simulink model "sampleModel1726"  (R2023a)
settings: Solver=VariableStepAuto  StartTime=0.0  StopTime=10.0  RelTol=1e-3
libraries: hdlsllib x4, simulink x2
settings Model: Creator=user1  LastModifiedBy=user1

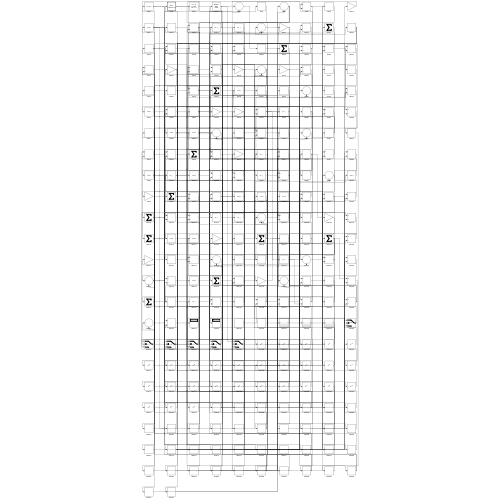
[thumbnail: Simulink's stored preview of the top-level diagram]
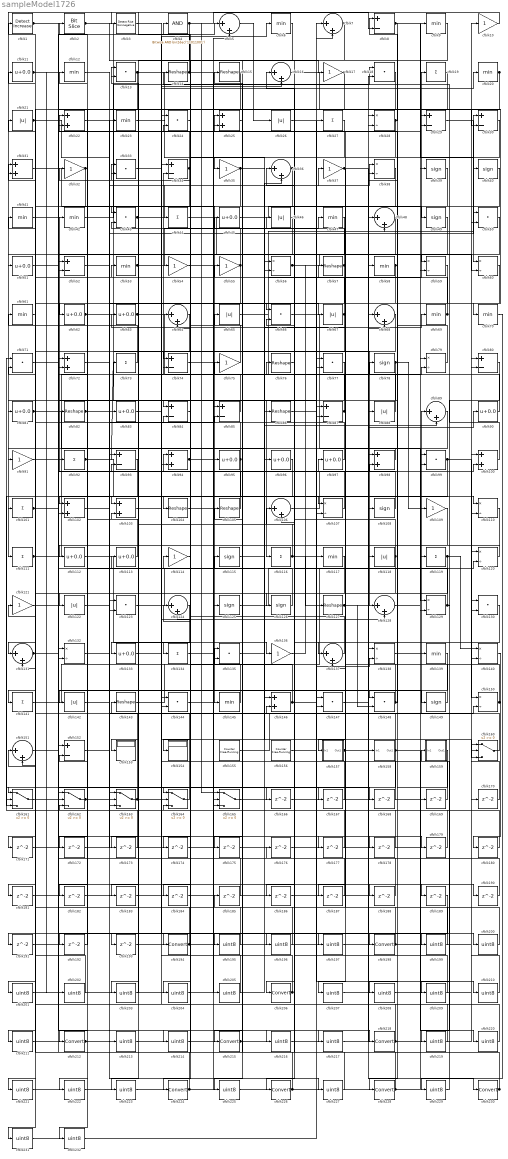
== system sampleModel1726 ==
  cfblk1 : simulink/Logic and Bit Operations/Detect Increase  vinit=0.0  OutDataTypeStr=boolean
      settings: LibrarySourceBlock=|
      | hdlsllib/Logic and Bit
      | Operations/Detect
      | Increase
  cfblk{10,17,32,35,37,54..55,75,91,109,114,121,136} (13 alike) : Gain
  cfblk{22,25,31,72,94,98,100,102..103,146} (10 alike) : Sum
  cfblk{19,27,44,73,92,101,111,116,119,134,141} (11 alike) : Sum  Inputs=+
  cfblk{14..15,57,76,82,86,104..105,127,143} (10 alike) : Reshape
  cfblk{5,7,16,36,48,64,68,89,106,124,128,131,137,151} (14 alike) : Sum  Inputs=|++
  cfblk{28,38,56,59..60,79,107,110,120,129,132,138,140,150} (14 alike) : Product  Inputs=*/  RndMeth=Zero  SaturateOnIntegerOverflow=on
  cfblk{39..40,49,78,108,115,125..126,149} (9 alike) : Signum
  cfblk{11,45,51,62..63,81,83,90,95..97,112..113,133} (14 alike) : Bias  Bias=0.0  SaturateOnIntegerOverflow=off
  cfblk{6,9,12,20,23,41..42,47,53,58,61,69..70,117,139,145} (16 alike) : MinMax
  cfblk{21,26,46,65,67,88,118,122,142} (9 alike) : Abs  SaturateOnIntegerOverflow=off
  cfblk{13,18,24,33,43,50,66,71,77,99,123,130,135,144,147..148} (16 alike) : DotProduct  OutDataTypeStr=Inherit: Inherit via internal rule
  cfblk{8,29..30,34,52,74,80,84..85,87,93,152} (12 alike) : Sum  Inputs=+-
  cfblk153 : Display
  cfblk154 : Display
  cfblk155 : hdlsllib/Sources/Counter Free-Running  NumBits=16  tsamp=-1
  cfblk156 : hdlsllib/Sources/Counter Free-Running  NumBits=16  tsamp=-1
  cfblk157 : Subsystem
      settings: LibrarySourceBlock=|
      | hdlsllib/Ports &
      | Subsystems/Subsystem
  cfblk158 : Subsystem
      settings: LibrarySourceBlock=|
      | hdlsllib/Ports &
      | Subsystems/Subsystem
  cfblk159 : Subsystem
      settings: LibrarySourceBlock=|
      | hdlsllib/Ports &
      | Subsystems/Subsystem
  cfblk{160..165} (6 alike) : Switch  SaturateOnIntegerOverflow=off  InputSameDT=off
  cfblk{166..193} (28 alike) : Delay  SampleTime=1
  cfblk{194,198,206,212,215,218,224,226,228,230} (10 alike) : DataTypeConversion  SaturateOnIntegerOverflow=off  RndMeth=Floor
  cfblk{195..197,199..205,207..211,213..214,216..217,219..223,225,227,229,231..232} (29 alike) : DataTypeConversion  OutDataTypeStr=uint8  SaturateOnIntegerOverflow=off  RndMeth=Floor
  cfblk2 : hdlsllib/Logic and Bit Operations/Bit Slice  lidx=7  ridx=0
  cfblk3 : hdlsllib/Logic and Bit Operations/Detect Rise Nonnegative  vinit=0  OutDataTypeStr=boolean
  cfblk4 : simulink/Logic and Bit Operations/Bitwise Operator  logicop=AND  UseBitMask=on  BitMask=bin2dec('11011001')  BitMaskRealWorld=Stored Integer
      settings: LibrarySourceBlock=|
      | hdlsllib/Logic and Bit
      | Operations/Bitwise
      | Operator
  wires:
  cfblk5/1 -> cfblk26/1
  cfblk119/1 -> cfblk140/1, cfblk126/1, cfblk137/2, cfblk131/1
  cfblk95/1 -> cfblk42/1, cfblk165/2
  cfblk2/1 -> cfblk116/1, cfblk17/1
  cfblk14/1 -> cfblk111/1, cfblk110/1
  cfblk36/1 -> cfblk122/1, cfblk125/1
  cfblk92/1 -> cfblk73/1, cfblk158/1(In1)
  cfblk107/1 -> cfblk72/1
  cfblk76/1 -> cfblk226/1
  cfblk63/1 -> cfblk30/1, cfblk16/2, cfblk160/3
  cfblk16/1 -> cfblk70/1
  cfblk62/1 -> cfblk128/1, cfblk50/1
  cfblk123/1 -> cfblk36/2
  cfblk31/1 -> cfblk145/1
  cfblk29/1 -> cfblk60/1
  cfblk126/1 -> cfblk2/1
  cfblk11/1 -> cfblk30/2, cfblk87/2, cfblk189/1, cfblk202/1
  cfblk155/1 -> cfblk89/1
  cfblk71/1 -> cfblk5/1
  cfblk112/1 -> cfblk136/1
  cfblk149/1 -> cfblk94/1
  cfblk41/1 -> cfblk60/2
  cfblk150/1 -> cfblk55/1, cfblk25/2
  cfblk147/1 -> cfblk230/1
  cfblk7/1 -> cfblk84/1, cfblk104/1, cfblk223/1
  cfblk105/1 -> cfblk53/1
  cfblk68/1 -> cfblk215/1
  cfblk135/1 -> cfblk89/2
  cfblk152/1 -> cfblk198/1
  cfblk158/1(Out1) -> cfblk143/1, cfblk161/3, cfblk220/1
  cfblk42/1 -> cfblk18/1
  cfblk111/1 -> cfblk34/2, cfblk98/2
  cfblk43/1 -> cfblk37/1, cfblk165/3
  cfblk30/1 -> cfblk35/1
  cfblk78/1 -> cfblk134/1, cfblk109/1
  cfblk27/1 -> cfblk224/1
  cfblk136/1 -> cfblk117/1
  cfblk65/1 -> cfblk19/1
  cfblk113/1 -> cfblk52/1
  cfblk106/1 -> cfblk10/1
  cfblk57/1 -> cfblk141/1, cfblk24/2
  cfblk32/1 -> cfblk171/1, cfblk172/1
  cfblk35/1 -> cfblk154/1, cfblk160/2
  cfblk67/1 -> cfblk163/3, cfblk81/1, cfblk31/2
  cfblk17/1 -> cfblk102/1, cfblk232/1
  cfblk13/1 -> cfblk56/2, cfblk192/1
  cfblk141/1 -> cfblk28/1
  cfblk45/1 -> cfblk49/1
  cfblk75/1 -> cfblk32/1
  cfblk12/1 -> cfblk194/1
  cfblk90/1 -> cfblk33/1
  cfblk69/1 -> cfblk15/1, cfblk11/1
  cfblk97/1 -> cfblk41/1
  cfblk98/1 -> cfblk91/1
  cfblk118/1 -> cfblk63/1, cfblk187/1
  cfblk82/1 -> cfblk38/2, cfblk227/1
  cfblk129/1 -> cfblk106/2, cfblk219/1
  cfblk163/1 -> cfblk72/2, cfblk100/2, cfblk131/2
  cfblk121/1 -> cfblk92/1
  cfblk56/1 -> cfblk59/1, cfblk127/1, cfblk148/1
  cfblk23/1 -> cfblk86/1
  cfblk64/1 -> cfblk132/2
  cfblk165/1 -> cfblk39/1
  cfblk21/1 -> cfblk102/2, cfblk93/1
  cfblk159/1(Out1) -> cfblk228/1
  cfblk115/1 -> cfblk69/1
  cfblk59/1 -> cfblk95/1
  cfblk6/1 -> cfblk85/1
  cfblk86/1 -> cfblk7/1
  cfblk145/1 -> cfblk4/1
  cfblk162/1 -> cfblk23/1, cfblk150/2
  cfblk47/1 -> cfblk101/1
  cfblk48/1 -> cfblk212/1
  cfblk100/1 -> cfblk14/1
  cfblk20/1 -> cfblk62/1, cfblk51/1, cfblk74/1
  cfblk4/1 -> cfblk133/1, cfblk8/2, cfblk165/1
  cfblk72/1 -> cfblk83/1
  cfblk84/1 -> cfblk164/1
  cfblk160/1 -> cfblk25/1
  cfblk116/1 -> cfblk78/1, cfblk33/2
  cfblk66/1 -> cfblk129/1
  cfblk89/1 -> cfblk161/1
  cfblk99/1 -> cfblk150/1, cfblk161/2
  cfblk96/1 -> cfblk103/1
  cfblk46/1 -> cfblk123/2
  cfblk125/1 -> cfblk119/1
  cfblk143/1 -> cfblk28/2
  cfblk151/1 -> cfblk218/1
  cfblk130/1 -> cfblk206/1
  cfblk44/1 -> cfblk118/1
  cfblk37/1 -> cfblk137/1, cfblk200/1
  cfblk15/1 -> cfblk43/1
  cfblk19/1 -> cfblk142/1
  cfblk22/1 -> cfblk67/1
  cfblk117/1 -> cfblk153/1
  cfblk55/1 -> cfblk64/2, cfblk43/2, cfblk173/1
  cfblk87/1 -> cfblk54/1, cfblk207/1
  cfblk110/1 -> cfblk140/2
  cfblk34/1 -> cfblk13/1, cfblk144/2
  cfblk164/1 -> cfblk71/2
  cfblk133/1 -> cfblk128/2
  cfblk128/1 -> cfblk29/1
  cfblk81/1 -> cfblk146/1, cfblk164/2
  cfblk131/1 -> cfblk29/2, cfblk115/1
  cfblk108/1 -> cfblk13/2
  cfblk138/1 -> cfblk139/1
  cfblk101/1 -> cfblk110/2, cfblk179/1
  cfblk8/1 -> cfblk40/1, cfblk208/1
  cfblk157/1(Out1) -> cfblk57/1, cfblk120/2
  cfblk120/1 -> cfblk112/1
  cfblk58/1 -> cfblk88/1, cfblk191/1
  cfblk85/1 -> cfblk44/1
  cfblk137/1 -> cfblk82/1
  cfblk102/1 -> cfblk107/1
  cfblk148/1 -> cfblk64/1, cfblk38/1
  cfblk127/1 -> cfblk90/1, cfblk148/2
  cfblk18/1 -> cfblk66/1
  cfblk122/1 -> cfblk85/2
  cfblk1/1 -> cfblk149/1, cfblk108/1
  cfblk79/1 -> cfblk22/1
  cfblk73/1 -> cfblk31/1
  cfblk33/1 -> cfblk6/1
  cfblk88/1 -> cfblk45/1
  cfblk146/1 -> cfblk135/1, cfblk138/2
  cfblk49/1 -> cfblk162/2
  cfblk94/1 -> cfblk79/2, cfblk107/2
  cfblk10/1 -> cfblk3/1
  cfblk28/1 -> cfblk8/1, cfblk184/1
  cfblk109/1 -> cfblk157/1(In1)
  cfblk53/1 -> cfblk47/1, cfblk20/1
  cfblk83/1 -> cfblk166/1
  cfblk166/1 -> cfblk79/1
  cfblk142/1 -> cfblk167/1
  cfblk167/1 -> cfblk34/1
  cfblk144/1 -> cfblk168/1
  cfblk168/1 -> cfblk66/2
  cfblk169/1 -> cfblk56/1
  cfblk170/1 -> cfblk100/1
  cfblk171/1 -> cfblk163/2
  cfblk172/1 -> cfblk59/2
  cfblk173/1 -> cfblk71/1
  cfblk114/1 -> cfblk174/1
  cfblk174/1 -> cfblk7/2
  cfblk60/1 -> cfblk175/1
  cfblk175/1 -> cfblk129/2
  cfblk176/1 -> cfblk138/1
  cfblk74/1 -> cfblk177/1
  cfblk177/1 -> cfblk36/1
  cfblk103/1 -> cfblk178/1
  cfblk178/1 -> cfblk123/1
  cfblk179/1 -> cfblk1/1
  cfblk140/1 -> cfblk180/1
  cfblk180/1 -> cfblk163/1
  cfblk50/1 -> cfblk181/1
  cfblk181/1 -> cfblk94/2
  cfblk93/1 -> cfblk182/1
  cfblk39/1 -> cfblk183/1
  cfblk183/1 -> cfblk18/2
  cfblk184/1 -> cfblk84/2
  cfblk185/1 -> cfblk164/3
  cfblk38/1 -> cfblk186/1
  cfblk186/1 -> cfblk16/1
  cfblk187/1 -> cfblk162/3
  cfblk134/1 -> cfblk188/1
  cfblk188/1 -> cfblk106/1
  cfblk104/1 -> cfblk190/1
  cfblk190/1 -> cfblk162/1
  cfblk191/1 -> cfblk52/2
  cfblk192/1 -> cfblk22/2
  cfblk91/1 -> cfblk193/1
  cfblk193/1 -> cfblk98/1
  cfblk194/1 -> cfblk120/1, cfblk5/2, cfblk113/1
  cfblk3/1 -> cfblk195/1
  cfblk195/1 -> cfblk12/1
  cfblk9/1 -> cfblk196/1
  cfblk196/1 -> cfblk21/1
  cfblk51/1 -> cfblk197/1
  cfblk197/1 -> cfblk9/1
  cfblk198/1 -> cfblk93/2, cfblk97/1
  cfblk156/1 -> cfblk199/1
  cfblk199/1 -> cfblk152/1
  cfblk200/1 -> cfblk152/2
  cfblk61/1 -> cfblk201/1
  cfblk201/1 -> cfblk96/1
  cfblk202/1 -> cfblk61/1
  cfblk124/1 -> cfblk203/1
  cfblk203/1 -> cfblk103/2
  cfblk24/1 -> cfblk204/1
  cfblk204/1 -> cfblk124/1
  cfblk54/1 -> cfblk205/1
  cfblk205/1 -> cfblk124/2
  cfblk206/1 -> cfblk105/1, cfblk24/1
  cfblk207/1 -> cfblk130/1
  cfblk208/1 -> cfblk130/2
  cfblk80/1 -> cfblk209/1
  cfblk209/1 -> cfblk46/1
  cfblk26/1 -> cfblk210/1
  cfblk210/1 -> cfblk80/1
  cfblk189/1 -> cfblk211/1
  cfblk211/1 -> cfblk80/2
  cfblk212/1 -> cfblk87/1, cfblk50/2, cfblk99/2, cfblk160/1, cfblk58/1
  cfblk52/1 -> cfblk213/1
  cfblk213/1 -> cfblk48/1
  cfblk182/1 -> cfblk214/1
  cfblk214/1 -> cfblk48/2
  cfblk215/1 -> cfblk170/1, cfblk169/1
  cfblk161/1 -> cfblk216/1
  cfblk216/1 -> cfblk68/1
  cfblk132/1 -> cfblk217/1
  cfblk217/1 -> cfblk68/2
  cfblk218/1 -> cfblk144/1, cfblk65/1
  cfblk219/1 -> cfblk151/1
  cfblk220/1 -> cfblk151/2
  cfblk77/1 -> cfblk221/1
  cfblk221/1 -> cfblk99/1
  cfblk139/1 -> cfblk222/1
  cfblk222/1 -> cfblk77/1
  cfblk223/1 -> cfblk77/2
  cfblk224/1 -> cfblk135/2, cfblk132/1
  cfblk25/1 -> cfblk225/1
  cfblk225/1 -> cfblk27/1
  cfblk226/1 -> cfblk185/1, cfblk121/1, cfblk114/1
  cfblk227/1 -> cfblk76/1
  cfblk228/1 -> cfblk146/2, cfblk75/1
  cfblk70/1 -> cfblk229/1
  cfblk229/1 -> cfblk159/1(In1)
  cfblk230/1 -> cfblk176/1, cfblk74/2
  cfblk40/1 -> cfblk231/1
  cfblk231/1 -> cfblk147/1
  cfblk232/1 -> cfblk147/2

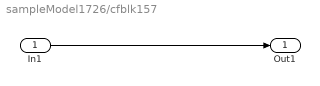
== system sampleModel1726/cfblk157 ==
  In1 : Inport
  Out1 : Outport
  wires:
  In1/1 -> Out1/1

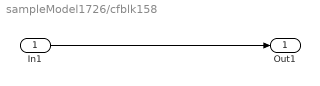
== system sampleModel1726/cfblk158 ==
  In1 : Inport
  Out1 : Outport
  wires:
  In1/1 -> Out1/1

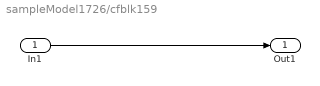
== system sampleModel1726/cfblk159 ==
  In1 : Inport
  Out1 : Outport
  wires:
  In1/1 -> Out1/1
